simulink model "opentopicSoftwareslx"  (R2024a)
settings: Solver=FixedStepAuto  StartTime=0.0  StopTime=inf  FixedStep=0.01  RelTol=1e-3
undefined symbols (not defined in the file or in its folder): LF
libraries: instrumentseriallib x3, simulink x2, hdlsllib x1
settings Model: Creator=tanawatp  LastModifiedBy=tanawatp

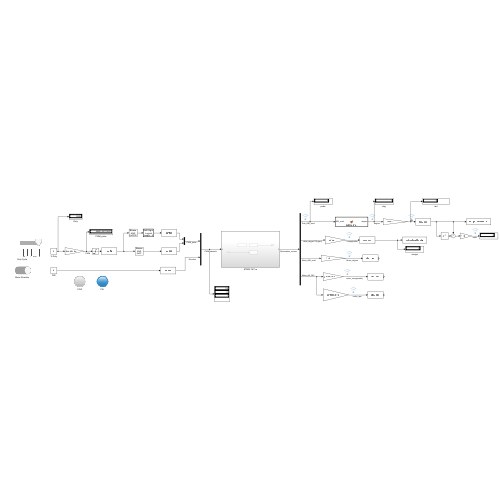
[thumbnail: Simulink's stored preview of the top-level diagram]
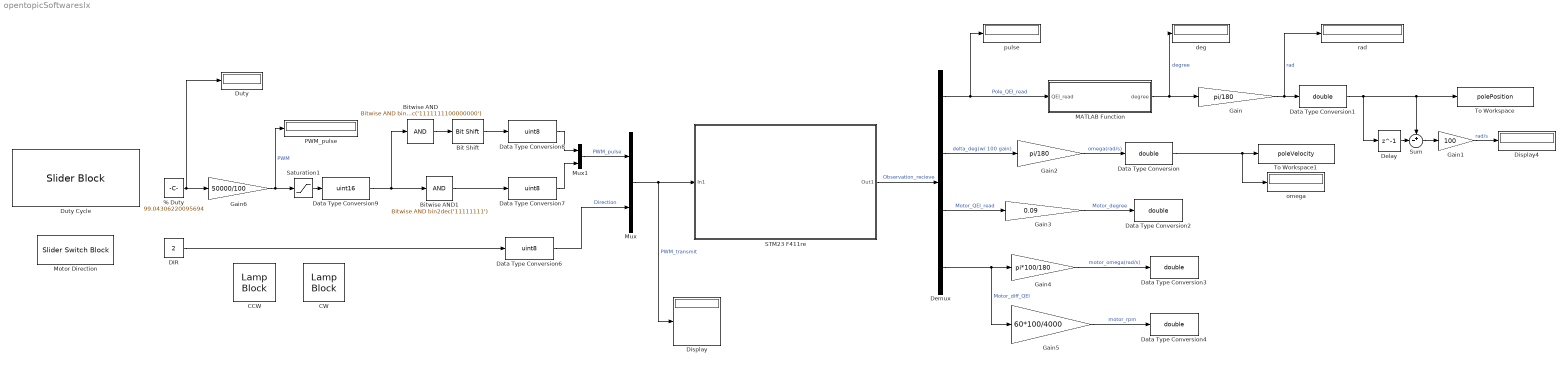
== system opentopicSoftwareslx ==
  % Duty : Constant  Value=99.04306220095694
  Bit Shift : hdlsllib/Logic and Bit Operations/Bit Shift  mode=Shift Right Logical  N=8
  Bitwise AND : simulink/Logic and Bit Operations/Bitwise Operator  logicop=AND  UseBitMask=on  BitMask=bin2dec('1111111100000000')  BitMaskRealWorld=Stored Integer
  Bitwise AND1 : simulink/Logic and Bit Operations/Bitwise Operator  logicop=AND  UseBitMask=on  BitMask=bin2dec('11111111')  BitMaskRealWorld=Stored Integer
  CCW : LampBlock  LabelPosition=Hide
  CW : LampBlock  LabelPosition=Hide
  "DIR " : Constant  Value=2
  Data Type Conversion{,1..4} (5 alike) : DataTypeConversion  OutDataTypeStr=double  SaturateOnIntegerOverflow=off  RndMeth=Floor
  Data Type Conversion6 : DataTypeConversion  OutDataTypeStr=uint8  SaturateOnIntegerOverflow=off  RndMeth=Floor
  Data Type Conversion7 : DataTypeConversion  OutDataTypeStr=uint8  SaturateOnIntegerOverflow=off  RndMeth=Floor
  Data Type Conversion8 : DataTypeConversion  OutDataTypeStr=uint8  SaturateOnIntegerOverflow=off  RndMeth=Floor
  Data Type Conversion9 : DataTypeConversion  OutDataTypeStr=uint16  SaturateOnIntegerOverflow=off  RndMeth=Floor
  Delay : Delay  DelayLength=1
  Demux : Demux
  Display : Display
  Display4 : Display
  Duty : Display
      settings: Decimation=2
  Duty Cycle : SliderBlock  LabelPosition=Hide
  Gain : Gain  Gain=pi/180  OutDataTypeStr=half
  Gain1 : Gain  Gain=100
  Gain2 : Gain  Gain=pi/180
  Gain3 : Gain  Gain=0.09  OutDataTypeStr=half
  Gain4 : Gain  Gain=pi*100/180
  Gain5 : Gain  Gain=60*100/4000
  Gain6 : Gain  Gain=50000/100
  MATLAB Function : MATLAB Function  TreatAsAtomicUnit=on
  Motor Direction : SliderSwitchBlock  LabelPosition=Hide
      settings: Values={{'CCW', 'CW'}, [1 2]}
  Mux : Mux  Inputs=2
  Mux1 : Mux  Inputs=2
  PWM_pulse : Display
      settings: Decimation=2
  STM23 F411re : Subsystem
  Saturation1 : Saturate  UpperLimit=50000  LowerLimit=5
  Sum : Sum  Inputs=+-|
  To Workspace : ToWorkspace  VariableName=polePosition  SaveFormat=Timeseries  SampleTime=-1
  To Workspace1 : ToWorkspace  VariableName=poleVelocity  SaveFormat=Timeseries  SampleTime=-1
  deg : Display
      settings: Decimation=4
  omega : Display
  pulse : Display
  rad : Display
      settings: Decimation=4
  wires:
  Gain4/1 -> Data Type Conversion3/1  "motor_omega(rad/s)"
  Demux/4 -> Gain5/1, Gain4/1  "Motor_diff_QEI"
  Delay/1 -> Sum/2
  Sum/1 -> Gain1/1
  Gain1/1 -> Display4/1  "rad/s"
  Gain5/1 -> Data Type Conversion4/1  "motor_rpm"
  Gain3/1 -> Data Type Conversion2/1  "Motor_degree"
  Data Type Conversion/1 -> To Workspace1/1, omega/1
  MATLAB Function/1(degree) -> deg/1, Gain/1  "degree"
  Demux/3 -> Gain3/1  "Motor_QEI_read"
  Data Type Conversion1/1 -> Sum/1, To Workspace/1, Delay/1
  Gain/1 -> Data Type Conversion1/1, rad/1  "rad"
  Gain2/1 -> Data Type Conversion/1  "omega(rad/s)"
  Demux/1 -> pulse/1, MATLAB Function/1(QEI_read)  "Pole_QEI_read"
  Demux/2 -> Gain2/1  "delta_deg(w/ 100 gain)"
  Data Type Conversion6/1 -> Mux/2  "Direction"
  "DIR "/1 -> Data Type Conversion6/1
  Data Type Conversion9/1 -> Bitwise AND1/1, Bitwise AND/1
  Data Type Conversion8/1 -> Mux1/1
  Bitwise AND1/1 -> Data Type Conversion7/1
  Mux1/1 -> Mux/1  "PWM_pulse"
  Data Type Conversion7/1 -> Mux1/2
  Saturation1/1 -> Data Type Conversion9/1
  Bit Shift/1 -> Data Type Conversion8/1
  Bitwise AND/1 -> Bit Shift/1
  % Duty/1 -> Duty/1, Gain6/1
  Gain6/1 -> PWM_pulse/1, Saturation1/1  "PWM"
  Mux/1 -> STM23 F411re/1(In1), Display/1  "PWM_transmit"
  STM23 F411re/1(Out1) -> Demux/1  "Observation_recieve"

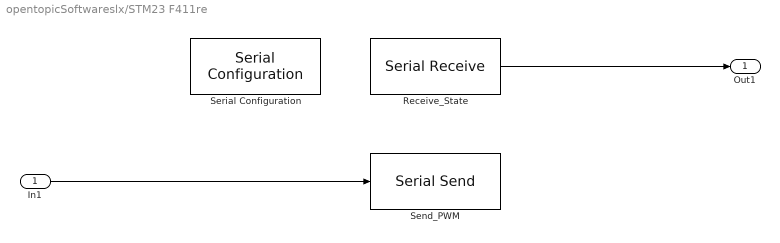
== system opentopicSoftwareslx/STM23 F411re ==
  In1 : Inport
  Receive_State : instrumentseriallib/Serial Receive  Priority=1  PortSel=COM6  Port=COM6  ComPort=COM6  DataType=int16  SaveDataType=uint8  ToggleHeader=on  Header=[61]  ToggleDataSize=on  DataSize=[4]  ToggleTerminator=on  Terminator=LF ('\n')  CustomTerminator=[]  InputFormat=Column major  EnableBlockingMode=on  ActionDataUnavailable=Output last received value  ActionWhenDataUnavailable=Output last received value  CustomValue=0  SampleTime=-1  SimulateUsing=Interpreted execution  BlockInModel=on  aMode=1
  Send_PWM : instrumentseriallib/Serial Send  Priority=1  PortSel=COM6  Port=COM6  ComPort=COM6  Header=[62]  Terminator=<none>  CustomTerminator=[123]  EnableBlockingMode=on  SimulateUsing=Interpreted execution  BlockInModel=on  aMode=1
  Serial Configuration : instrumentseriallib/Serial Configuration  Priority=-200000  PortSel=COM6  Port=COM6  ComPort=COM6  BaudRate=115200  DataBits=8  Parity=none  StopBits=1  ByteOrder=little-endian  FlowControl=none  Timeout=10  SimulateUsing=Interpreted execution  BlockInModel=on  aMode=1
  Out1 : Outport
  wires:
  Receive_State/1 -> Out1/1
  In1/1 -> Send_PWM/1

== matlab function opentopicSoftwareslx/MATLAB Function ==
  data: QEI_read input; degree output
function degree = poleDegree(QEI_read)
QEI_read = double(QEI_read);
if (QEI_read<=2000)
    degree = QEI_read*0.09;
else
    degree = (QEI_read-4000)*0.09;
end
